simulink model "rigidBody_lib_example"  (R2018b)
settings: Solver=VariableStepAuto  StartTime=0.0  StopTime=10.0  RelTol=1e-3
libraries: rigidBody_lib x4, axes_transformation_lib x1
settings Model: Creator=yannic  LastModifiedBy=yannic

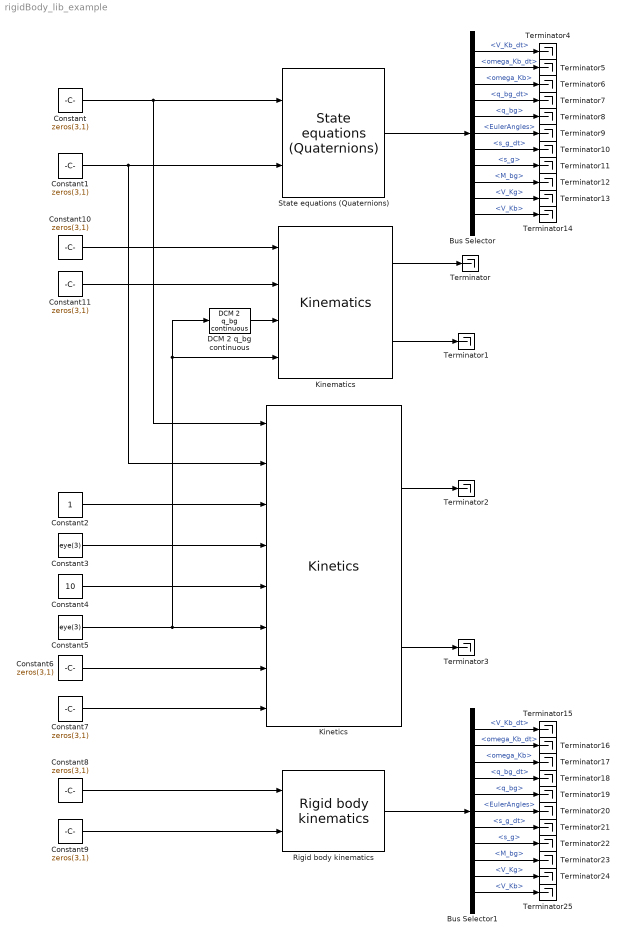
== system rigidBody_lib_example ==
  Bus Selector : BusSelector  OutputSignals=V_Kb_dt,omega_Kb_dt,omega_Kb,q_bg_dt,q_bg,EulerAngles,s_g_dt,s_g,M_bg,V_Kg,V_Kb
  Bus Selector1 : BusSelector  OutputSignals=V_Kb_dt,omega_Kb_dt,omega_Kb,q_bg_dt,q_bg,EulerAngles,s_g_dt,s_g,M_bg,V_Kg,V_Kb
  Constant{,1,6..11} (8 alike) : Constant  Value=zeros(3,1)
  Constant2 : Constant
  Constant3 : Constant  Value=eye(3)
  Constant4 : Constant  Value=10
  Constant5 : Constant  Value=eye(3)
  DCM 2 q_bg continuous : axes_transformation_lib/DCM 2 q_bg continuous
      settings: SourceProductName=LADAC
  Kinematics : rigidBody_lib/Kinematics
      settings: SourceProductName=LADAC
  Kinetics : rigidBody_lib/Kinetics
      settings: SourceProductName=LADAC
  Rigid body kinematics : rigidBody_lib/Rigid body kinematics  omega_Kb_0=[0;0;0]  q_bg_0=[1;0;0;0]  V_Kb_0=[0;0;0]  s_g_0=[0;0;0]
      settings: SourceProductName=LADAC
  State equations (Quaternions) : rigidBody_lib/State equations (Quaternions)  m=1  I=eye(3)  is_g_checked=off  g=10  omega_Kb_0=[0,0,0]'  q_bg_0=[1,0,0,0]'  V_Kb_0=[0,0,0]'  s_g_0=[0,0,0]'
      settings: SourceProductName=LADAC
  Terminator{,1..25} (26 alike) : Terminator
  wires:
  Constant/1 -> Kinetics/1, State equations (Quaternions)/1
  Constant1/1 -> Kinetics/2, State equations (Quaternions)/2
  Constant2/1 -> Kinetics/3
  Constant3/1 -> Kinetics/4
  Constant4/1 -> Kinetics/5
  Constant5/1 -> DCM 2 q_bg continuous/1, Kinematics/4, Kinetics/6
  Constant6/1 -> Kinetics/7
  Constant7/1 -> Kinetics/8
  Constant8/1 -> Rigid body kinematics/1
  Constant9/1 -> Rigid body kinematics/2
  State equations (Quaternions)/1 -> Bus Selector/1
  Rigid body kinematics/1 -> Bus Selector1/1
  Kinematics/1 -> Terminator/1
  Kinematics/2 -> Terminator1/1
  Kinetics/1 -> Terminator2/1
  Kinetics/2 -> Terminator3/1
  Bus Selector/1 -> Terminator4/1  "<V_Kb_dt>"
  Bus Selector/2 -> Terminator5/1  "<omega_Kb_dt>"
  Bus Selector/3 -> Terminator6/1  "<omega_Kb>"
  Bus Selector/4 -> Terminator7/1  "<q_bg_dt>"
  Bus Selector/5 -> Terminator8/1  "<q_bg>"
  Bus Selector/6 -> Terminator9/1  "<EulerAngles>"
  Bus Selector/7 -> Terminator10/1  "<s_g_dt>"
  Bus Selector/8 -> Terminator11/1  "<s_g>"
  Bus Selector/9 -> Terminator12/1  "<M_bg>"
  Bus Selector/10 -> Terminator13/1  "<V_Kg>"
  Bus Selector/11 -> Terminator14/1  "<V_Kb>"
  Bus Selector1/1 -> Terminator15/1  "<V_Kb_dt>"
  Bus Selector1/2 -> Terminator16/1  "<omega_Kb_dt>"
  Bus Selector1/3 -> Terminator17/1  "<omega_Kb>"
  Bus Selector1/4 -> Terminator18/1  "<q_bg_dt>"
  Bus Selector1/5 -> Terminator19/1  "<q_bg>"
  Bus Selector1/6 -> Terminator20/1  "<EulerAngles>"
  Bus Selector1/7 -> Terminator21/1  "<s_g_dt>"
  Bus Selector1/8 -> Terminator22/1  "<s_g>"
  Bus Selector1/9 -> Terminator23/1  "<M_bg>"
  Bus Selector1/10 -> Terminator24/1  "<V_Kg>"
  Bus Selector1/11 -> Terminator25/1  "<V_Kb>"
  Constant10/1 -> Kinematics/1
  Constant11/1 -> Kinematics/2
  DCM 2 q_bg continuous/1 -> Kinematics/3
